simulink model "butterfly_dsp48e_6slice"  (R2012b)
settings: Solver=ode45  StartTime=0.0  StopTime=1999  RelTol=1e-3
libraries: xbsIndex_r4 x255, simulink x8, casper_library_misc x6
(part 1 of 2)
settings Model: Creator=sgowda  LastModifiedBy=sgowda

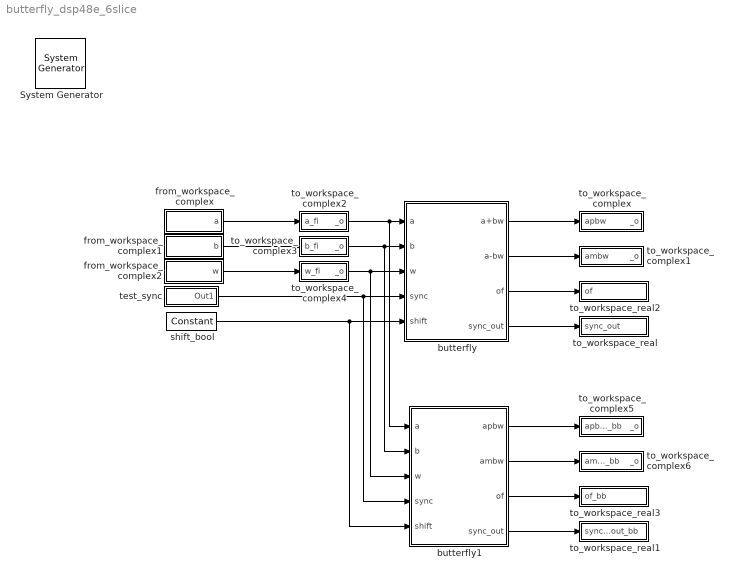
== system butterfly_dsp48e_6slice ==
  " System Generator" : xbsIndex_r4/ System Generator  Tag=genX  xilinxfamily=Kintex7  part=xc7k325t  speed=-3  package=fbg676  synthesis_tool=XST  clock_wrapper=Clock Enables  directory=./netlist  proj_type=Project Navigator  Synth_file=XST Defaults  Impl_file=ISE Defaults  testbench=off  simulink_period=1  sysclk_period=10  dcm_input_clock_period=10  incr_netlist=off  trim_vbits=Everywhere in SubSystem  dbl_ovrd=According to Block Masks  core_generation=According to Block Masks  run_coregen=off  deprecated_control=off  eval_field=0  block_type=sysgen
  butterfly : Subsystem
      settings: AttributesFormatString=|
      | twiddle_general_dsp48e
      | coeffs in slices
      | Bit growth:0
  butterfly1 : Subsystem
  from_workspace_complex : Subsystem  mask{var_name=a, n_bits=18, bin_pt=17, quantization=Truncate, overflow=Wrap, arith_type=Signed  (2's comp)}
      mask prompts: var_name "Workspace variable name"; n_bits "# of bits"; bin_pt "Binary Point"; arith_type "Arithmetic type"
      mask init:
      | config.source = str2func('mat_input_data_cplx_init_xblock');
      | config.toplevel = gcb();
      | xBlock(config, {config.toplevel, 'var_name', var_name, ...
      |     'n_bits', n_bits, 'bin_pt', bin_pt, 'quantization', quantization, ...
      |     'overflow', overflow, 'arith_type', arith_type});
      mask TypeOptions quantization: Truncate | Round  (unbiased: +/- Inf) | Round  (unbiased: Even Values)
      mask TypeOptions overflow: Wrap | Saturate | Flag as error
      mask TypeOptions arith_type: Signed  (2's comp) | Boolean | Unsigned
  from_workspace_complex1 : Subsystem  mask{var_name=b, n_bits=18, bin_pt=17, quantization=Truncate, overflow=Wrap, arith_type=Signed  (2's comp)}
      mask prompts: var_name "Workspace variable name"; n_bits "# of bits"; bin_pt "Binary Point"; arith_type "Arithmetic type"
      mask init: same as butterfly_dsp48e_6slice/from_workspace_complex
      mask TypeOptions quantization: Truncate | Round  (unbiased: +/- Inf) | Round  (unbiased: Even Values)
      mask TypeOptions overflow: Wrap | Saturate | Flag as error
      mask TypeOptions arith_type: Signed  (2's comp) | Boolean | Unsigned
  from_workspace_complex2 : Subsystem  mask{var_name=w, n_bits=18, bin_pt=17, quantization=Truncate, overflow=Wrap, arith_type=Signed  (2's comp)}
      mask prompts: var_name "Workspace variable name"; n_bits "# of bits"; bin_pt "Binary Point"; arith_type "Arithmetic type"
      mask init: same as butterfly_dsp48e_6slice/from_workspace_complex
      mask TypeOptions quantization: Truncate | Round  (unbiased: +/- Inf) | Round  (unbiased: Even Values)
      mask TypeOptions overflow: Wrap | Saturate | Flag as error
      mask TypeOptions arith_type: Signed  (2's comp) | Boolean | Unsigned
  shift_bool : xbsIndex_r4/Constant  const=0  gui_display_data_type=Boolean  arith_type=Boolean  n_bits=32  bin_pt=0  preci_type=Single  exp_width=8  frac_width=24  explicit_period=on  period=1  equ=P=C  opselect=C  inp2=PCIN>>17  opr=+  inp1=P  carry=CIN  dbl_ovrd=off  block_type=constant
  test_sync : Subsystem
  to_workspace_complex : Subsystem  mask{var_name=apbw, n_bits=18, bin_pt=17}
      mask prompts: var_name "Workspace variable name"; n_bits "# of bits"; bin_pt "Binary Point"
      mask init:
      | config.source = str2func('mat_output_data_cplx_init_xblock');
      | config.toplevel = gcb();
      | xBlock(config, {config.toplevel, 'var_name', var_name, ...
      |     'n_bits', n_bits, 'bin_pt', bin_pt})
  to_workspace_complex1 : Subsystem  mask{var_name=ambw, n_bits=18, bin_pt=17}
      mask prompts: var_name "Workspace variable name"; n_bits "# of bits"; bin_pt "Binary Point"
      mask init:
      | config.source = str2func('mat_output_data_cplx_init_xblock');
      | config.toplevel = gcb();
      | xBlock(config, {config.toplevel, 'var_name', var_name, ...
      |     'n_bits', n_bits, 'bin_pt', bin_pt})
  to_workspace_complex2 : Subsystem  mask{var_name=a_fi, n_bits=18, bin_pt=17}
      mask prompts: var_name "Workspace variable name"; n_bits "# of bits"; bin_pt "Binary Point"
      mask init:
      | config.source = str2func('mat_output_data_cplx_init_xblock');
      | config.toplevel = gcb();
      | xBlock(config, {config.toplevel, 'var_name', var_name, ...
      |     'n_bits', n_bits, 'bin_pt', bin_pt});
  to_workspace_complex3 : Subsystem  mask{var_name=b_fi, n_bits=18, bin_pt=17}
      mask prompts: var_name "Workspace variable name"; n_bits "# of bits"; bin_pt "Binary Point"
      mask init:
      | config.source = str2func('mat_output_data_cplx_init_xblock');
      | config.toplevel = gcb();
      | xBlock(config, {config.toplevel, 'var_name', var_name, ...
      |     'n_bits', n_bits, 'bin_pt', bin_pt});
  to_workspace_complex4 : Subsystem  mask{var_name=w_fi, n_bits=18, bin_pt=17}
      mask prompts: var_name "Workspace variable name"; n_bits "# of bits"; bin_pt "Binary Point"
      mask init:
      | config.source = str2func('mat_output_data_cplx_init_xblock');
      | config.toplevel = gcb();
      | xBlock(config, {config.toplevel, 'var_name', var_name, ...
      |     'n_bits', n_bits, 'bin_pt', bin_pt});
  to_workspace_complex5 : Subsystem  mask{var_name=apbw_bb, n_bits=18, bin_pt=17}
      mask prompts: var_name "Workspace variable name"; n_bits "# of bits"; bin_pt "Binary Point"
      mask init:
      | config.source = str2func('mat_output_data_cplx_init_xblock');
      | config.toplevel = gcb();
      | xBlock(config, {config.toplevel, 'var_name', var_name, ...
      |     'n_bits', n_bits, 'bin_pt', bin_pt})
  to_workspace_complex6 : Subsystem  mask{var_name=ambw_bb, n_bits=18, bin_pt=17}
      mask prompts: var_name "Workspace variable name"; n_bits "# of bits"; bin_pt "Binary Point"
      mask init:
      | config.source = str2func('mat_output_data_cplx_init_xblock');
      | config.toplevel = gcb();
      | xBlock(config, {config.toplevel, 'var_name', var_name, ...
      |     'n_bits', n_bits, 'bin_pt', bin_pt})
  to_workspace_real : Subsystem  mask{var_name=sync_out}
      mask prompts: var_name "Workspace variable name"
      mask init:
      | config.source = str2func('mat_output_data_init_xblock');
      | config.toplevel = gcb();
      | xBlock(config, {config.toplevel, 'var_name', var_name});
  to_workspace_real1 : Subsystem  mask{var_name=sync_out_bb}
      mask prompts: var_name "Workspace variable name"
      mask init:
      | config.source = str2func('mat_output_data_init_xblock');
      | config.toplevel = gcb();
      | xBlock(config, {config.toplevel, 'var_name', var_name});
  to_workspace_real2 : Subsystem  mask{var_name=of}
      mask prompts: var_name "Workspace variable name"
      mask init:
      | config.source = str2func('mat_output_data_init_xblock');
      | config.toplevel = gcb();
      | xBlock(config, {config.toplevel, 'var_name', var_name});
  to_workspace_real3 : Subsystem  mask{var_name=of_bb}
      mask prompts: var_name "Workspace variable name"
      mask init:
      | config.source = str2func('mat_output_data_init_xblock');
      | config.toplevel = gcb();
      | xBlock(config, {config.toplevel, 'var_name', var_name});
  wires:
  shift_bool/1 -> butterfly/5(shift), butterfly1/5(shift)
  butterfly/1(a+bw) -> to_workspace_complex/1(apbw)
  butterfly/2(a-bw) -> to_workspace_complex1/1(ambw)
  butterfly/4(sync_out) -> to_workspace_real/1(sync_out)
  butterfly/3(of) -> to_workspace_real2/1(of)
  test_sync/1(Out1) -> butterfly1/4(sync), butterfly/4(sync)
  from_workspace_complex/1(a) -> to_workspace_complex2/1(a_fi)
  from_workspace_complex1/1(b) -> to_workspace_complex3/1(b_fi)
  from_workspace_complex2/1(w) -> to_workspace_complex4/1(w_fi)
  to_workspace_complex2/1(_o) -> butterfly1/1(a), butterfly/1(a)
  to_workspace_complex3/1(_o) -> butterfly1/2(b), butterfly/2(b)
  to_workspace_complex4/1(_o) -> butterfly/3(w), butterfly1/3(w)
  butterfly1/1(apbw) -> to_workspace_complex5/1(apbw_bb)
  butterfly1/2(ambw) -> to_workspace_complex6/1(ambw_bb)
  butterfly1/3(of) -> to_workspace_real3/1(of_bb)
  butterfly1/4(sync_out) -> to_workspace_real1/1(sync_out_bb)

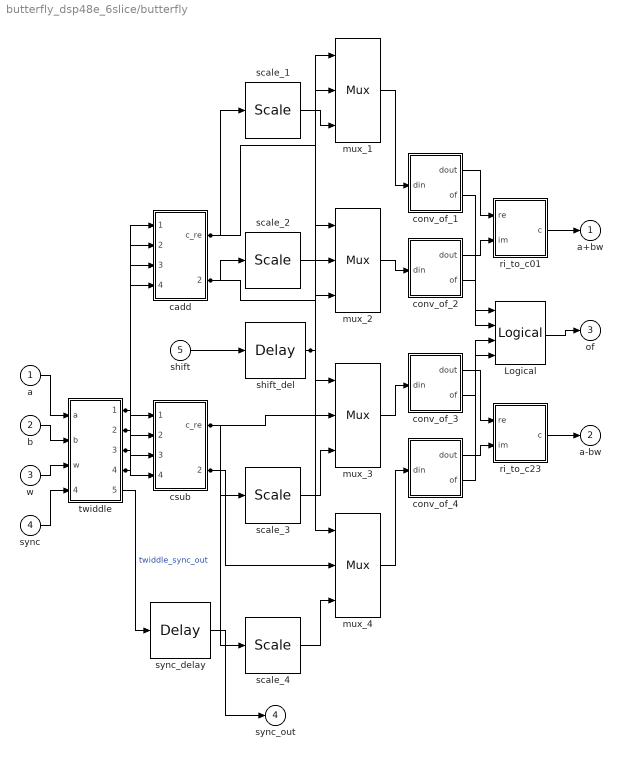
== system butterfly_dsp48e_6slice/butterfly ==
  a : Inport
  b : Inport  Port=2
  w : Inport  Port=3
  sync : Inport  Port=4
  shift : Inport  Port=5
  Logical : xbsIndex_r4/Logical  logical_function=OR  inputs=4  en=off  latency=0  precision=Full  arith_type=Unsigned  n_bits=16  bin_pt=0  align_bp=on  dbl_ovrd=off  block_type=logical
  cadd : Subsystem
  conv_of_1 : Subsystem
      settings: AttributesFormatString=[24,20]->[18,17]
  conv_of_2 : Subsystem
      settings: AttributesFormatString=[24,20]->[18,17]
  conv_of_3 : Subsystem
      settings: AttributesFormatString=[24,20]->[18,17]
  conv_of_4 : Subsystem
      settings: AttributesFormatString=[24,20]->[18,17]
  csub : Subsystem
  mux_{1..4} (4 alike) : xbsIndex_r4/Mux  inputs=2  en=off  latency=1  precision=Full  arith_type=Unsigned  n_bits=16  bin_pt=14  quantization=Truncate  overflow=Wrap  dbl_ovrd=off  block_type=mux
  ri_to_c01 : Subsystem
  ri_to_c23 : Subsystem
  scale_{1..4} (4 alike) : xbsIndex_r4/Scale  scale_factor=-1  dbl_ovrd=off  block_type=scale
  shift_del : xbsIndex_r4/Delay  rst=off  infoeditControl=Selection of Reset will increase slice count due to use of real FFs and instead of SRLs  en=off  latency=2  dbl_ovrd=off  reg_retiming=off  block_type=delay
  sync_delay : xbsIndex_r4/Delay  rst=off  infoeditControl=Selection of Reset will increase slice count due to use of real FFs and instead of SRLs  en=off  latency=4  dbl_ovrd=off  reg_retiming=on  block_type=delay
  twiddle : Subsystem
      settings: AttributesFormatString=|
      | data=(18,17)
      | coeffs=(18,16)
      | Virtex5
      | (Round  (unbiased: +/- Inf),Wrap)
      | twiddle_general_dsp48e
  a+bw : Outport
  a-bw : Outport  Port=2
  of : Outport  Port=3
  sync_out : Outport  Port=4
  wires:
  twiddle/1(a_re) -> csub/1(a_re), cadd/1(a_re)
  twiddle/2(a_im) -> csub/2(a_im), cadd/2(a_im)
  twiddle/3(bw_re) -> csub/3(b_re), cadd/3(b_re)
  twiddle/4(bw_im) -> csub/4(b_im), cadd/4(b_im)
  cadd/1(c_re) -> mux_1/2, scale_1/1
  shift_del/1 -> mux_4/1, mux_3/1, mux_2/1, mux_1/1
  cadd/2(c_im) -> mux_2/2, scale_2/1
  csub/1(c_re) -> mux_3/2, scale_3/1
  csub/2(c_im) -> mux_4/2, scale_4/1
  sync_delay/1 -> sync_out/1
  twiddle/5(sync_out) -> sync_delay/1  "twiddle_sync_out"
  ri_to_c23/1(c) -> a-bw/1
  conv_of_4/1(dout) -> ri_to_c23/2(im)
  conv_of_3/1(dout) -> ri_to_c23/1(re)
  ri_to_c01/1(c) -> a+bw/1
  conv_of_2/1(dout) -> ri_to_c01/2(im)
  conv_of_1/1(dout) -> ri_to_c01/1(re)
  Logical/1 -> of/1
  conv_of_4/2(of) -> Logical/4
  conv_of_3/2(of) -> Logical/3
  conv_of_2/2(of) -> Logical/2
  conv_of_1/2(of) -> Logical/1
  mux_4/1 -> conv_of_4/1(din)
  scale_4/1 -> mux_4/3
  mux_3/1 -> conv_of_3/1(din)
  scale_3/1 -> mux_3/3
  mux_2/1 -> conv_of_2/1(din)
  scale_2/1 -> mux_2/3
  mux_1/1 -> conv_of_1/1(din)
  scale_1/1 -> mux_1/3
  shift/1 -> shift_del/1
  sync/1 -> twiddle/4(sync)
  w/1 -> twiddle/3(w)
  b/1 -> twiddle/2(b)
  a/1 -> twiddle/1(a)

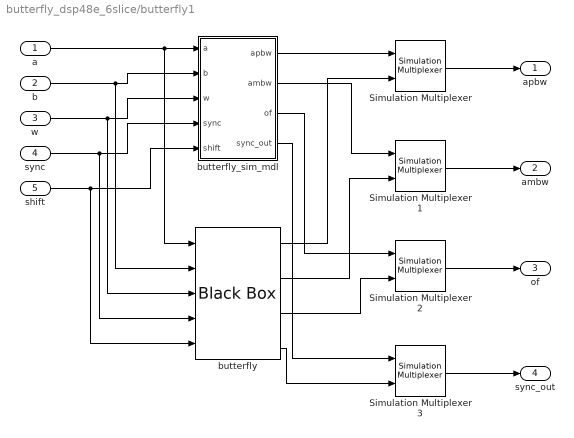
== system butterfly_dsp48e_6slice/butterfly1 ==
  a : Inport
  b : Inport  Port=2
  w : Inport  Port=3
  sync : Inport  Port=4
  shift : Inport  Port=5
  Simulation Multiplexer{,1..3} (4 alike) : xbsIndex_r4/Simulation Multiplexer  sim_sel=1  hw_sel=2  block_type=simmux
      settings: infoedit="Distinguish input subsystems as \"simulation only\" and \"generation only\".  The input specified For Simulation will be used during Simulink simulation.  The input specified For Generation will be used during code generation.  This block will typically be used on the output of a HW Co-Simulation, Black Box, or ModelSim subsystem.<br><br>Hardware Notes: This block costs nothing."
  butterfly : xbsIndex_r4/Black Box  init_code=butterfly_dsp48e_6slice_blackbox_config  sim_method=Inactive  verbose=off  block_type=blackbox2
  butterfly_sim_mdl : Subsystem
  apbw : Outport
  ambw : Outport  Port=2
  of : Outport  Port=3
  sync_out : Outport  Port=4
  wires:
  butterfly/2 -> Simulation Multiplexer1/2
  Simulation Multiplexer1/1 -> ambw/1
  Simulation Multiplexer/1 -> apbw/1
  butterfly_sim_mdl/1(apbw) -> Simulation Multiplexer/1
  butterfly_sim_mdl/3(of) -> Simulation Multiplexer2/1
  butterfly_sim_mdl/2(ambw) -> Simulation Multiplexer1/1
  butterfly/4 -> Simulation Multiplexer3/2
  b/1 -> butterfly/2, butterfly_sim_mdl/2(b)
  a/1 -> butterfly/1, butterfly_sim_mdl/1(a)
  w/1 -> butterfly/3, butterfly_sim_mdl/3(w)
  sync/1 -> butterfly/4, butterfly_sim_mdl/4(sync)
  butterfly/3 -> Simulation Multiplexer2/2
  butterfly_sim_mdl/4(sync_out) -> Simulation Multiplexer3/1
  butterfly/1 -> Simulation Multiplexer/2
  Simulation Multiplexer2/1 -> of/1
  Simulation Multiplexer3/1 -> sync_out/1
  shift/1 -> butterfly/5, butterfly_sim_mdl/5(shift)

== system butterfly_dsp48e_6slice/from_workspace_complex ==
  c_to_ri_simulink : ComplexToRealImag
  gateway_imag : xbsIndex_r4/Gateway In  gui_display_data_type=Fixed-point  arith_type="Signed  (2's comp)"  n_bits=18  bin_pt=17  preci_type=Single  exp_width=8  frac_width=24  quantization=Truncate  overflow=Wrap  period=1  dbl_ovrd=off  timing_constraint=None  locs_specified=off  LOCs={}  UseAsADC=off  ADCChannel='1'  inherit_from_input=off  hdl_port=on  block_type=gatewayin
  gateway_real : xbsIndex_r4/Gateway In  gui_display_data_type=Fixed-point  arith_type="Signed  (2's comp)"  n_bits=18  bin_pt=17  preci_type=Single  exp_width=8  frac_width=24  quantization=Truncate  overflow=Wrap  period=1  dbl_ovrd=off  timing_constraint=None  locs_specified=off  LOCs={}  UseAsADC=off  ADCChannel='1'  inherit_from_input=off  hdl_port=on  block_type=gatewayin
  ri_to_c : Subsystem
  workspace_var : FromWorkspace  VariableName=a  SampleTime=0
  a : Outport
  wires:
  ri_to_c/1(c) -> a/1
  gateway_imag/1 -> ri_to_c/2(im)
  gateway_real/1 -> ri_to_c/1(re)
  c_to_ri_simulink/2 -> gateway_imag/1
  c_to_ri_simulink/1 -> gateway_real/1
  workspace_var/1 -> c_to_ri_simulink/1

== system butterfly_dsp48e_6slice/from_workspace_complex1 ==
  c_to_ri_simulink : ComplexToRealImag
  gateway_imag : xbsIndex_r4/Gateway In  gui_display_data_type=Fixed-point  arith_type="Signed  (2's comp)"  n_bits=18  bin_pt=17  preci_type=Single  exp_width=8  frac_width=24  quantization=Truncate  overflow=Wrap  period=1  dbl_ovrd=off  timing_constraint=None  locs_specified=off  LOCs={}  UseAsADC=off  ADCChannel='1'  inherit_from_input=off  hdl_port=on  block_type=gatewayin
  gateway_real : xbsIndex_r4/Gateway In  gui_display_data_type=Fixed-point  arith_type="Signed  (2's comp)"  n_bits=18  bin_pt=17  preci_type=Single  exp_width=8  frac_width=24  quantization=Truncate  overflow=Wrap  period=1  dbl_ovrd=off  timing_constraint=None  locs_specified=off  LOCs={}  UseAsADC=off  ADCChannel='1'  inherit_from_input=off  hdl_port=on  block_type=gatewayin
  ri_to_c : Subsystem
  workspace_var : FromWorkspace  VariableName=b  SampleTime=0
  b : Outport
  wires:
  ri_to_c/1(c) -> b/1
  gateway_imag/1 -> ri_to_c/2(im)
  gateway_real/1 -> ri_to_c/1(re)
  c_to_ri_simulink/2 -> gateway_imag/1
  c_to_ri_simulink/1 -> gateway_real/1
  workspace_var/1 -> c_to_ri_simulink/1

== system butterfly_dsp48e_6slice/from_workspace_complex2 ==
  c_to_ri_simulink : ComplexToRealImag
  gateway_imag : xbsIndex_r4/Gateway In  gui_display_data_type=Fixed-point  arith_type="Signed  (2's comp)"  n_bits=18  bin_pt=17  preci_type=Single  exp_width=8  frac_width=24  quantization=Truncate  overflow=Wrap  period=1  dbl_ovrd=off  timing_constraint=None  locs_specified=off  LOCs={}  UseAsADC=off  ADCChannel='1'  inherit_from_input=off  hdl_port=on  block_type=gatewayin
  gateway_real : xbsIndex_r4/Gateway In  gui_display_data_type=Fixed-point  arith_type="Signed  (2's comp)"  n_bits=18  bin_pt=17  preci_type=Single  exp_width=8  frac_width=24  quantization=Truncate  overflow=Wrap  period=1  dbl_ovrd=off  timing_constraint=None  locs_specified=off  LOCs={}  UseAsADC=off  ADCChannel='1'  inherit_from_input=off  hdl_port=on  block_type=gatewayin
  ri_to_c : Subsystem
  workspace_var : FromWorkspace  VariableName=w  SampleTime=0
  w : Outport
  wires:
  ri_to_c/1(c) -> w/1
  gateway_imag/1 -> ri_to_c/2(im)
  gateway_real/1 -> ri_to_c/1(re)
  c_to_ri_simulink/2 -> gateway_imag/1
  c_to_ri_simulink/1 -> gateway_real/1
  workspace_var/1 -> c_to_ri_simulink/1

== system butterfly_dsp48e_6slice/test_sync ==
  Constant1 : xbsIndex_r4/Constant  const=1  gui_display_data_type=Boolean  arith_type=Boolean  n_bits=16  bin_pt=14  preci_type=Single  exp_width=8  frac_width=24  explicit_period=on  period=1  equ=P=C  opselect=C  inp2=PCIN>>17  opr=+  inp1=P  carry=CIN  dbl_ovrd=off  block_type=constant
  edge_detect : casper_library_misc/edge_detect  edge=Rising  polarity=Active High  x_in=[0 0.08 0.08 0.16 0.16 0.24 0.24 0.32 0.32 0.4]  y_in="[-1 -1  1  1  1  1  1  1  1  1]"  x_out=[0.6 0.68 0.68 0.76 0.76 0.84 0.84 0.92 0.92 1]  y_out="[-1 -1  1  1 -1 -1 -1 -1 -1 -1]"
  Out1 : Outport
  wires:
  edge_detect/1 -> Out1/1
  Constant1/1 -> edge_detect/1

== system butterfly_dsp48e_6slice/to_workspace_complex ==
  apbw : Inport
  c_to_ri : Subsystem
  imag_gateway : xbsIndex_r4/Gateway Out  inherit_from_input=on  hdl_port=off  timing_constraint=None  locs_specified=off  LOCs={}  UseAsDAC=off  DACChannel='1'  block_type=gatewayout
  real_gateway : xbsIndex_r4/Gateway Out  inherit_from_input=on  hdl_port=off  timing_constraint=None  locs_specified=off  LOCs={}  UseAsDAC=off  DACChannel='1'  block_type=gatewayout
  ri_to_c : RealImagToComplex
  workspace_output : ToWorkspace  VariableName=apbw  SampleTime=-1
  _o : Outport
  wires:
  apbw/1 -> c_to_ri/1(c), _o/1
  ri_to_c/1 -> workspace_output/1  "cplx"
  imag_gateway/1 -> ri_to_c/2
  real_gateway/1 -> ri_to_c/1
  c_to_ri/2(im) -> imag_gateway/1  "c_to_ri_out2"
  c_to_ri/1(re) -> real_gateway/1  "c_to_ri_out1"

== system butterfly_dsp48e_6slice/to_workspace_complex1 ==
  ambw : Inport
  c_to_ri : Subsystem
  imag_gateway : xbsIndex_r4/Gateway Out  inherit_from_input=on  hdl_port=off  timing_constraint=None  locs_specified=off  LOCs={}  UseAsDAC=off  DACChannel='1'  block_type=gatewayout
  real_gateway : xbsIndex_r4/Gateway Out  inherit_from_input=on  hdl_port=off  timing_constraint=None  locs_specified=off  LOCs={}  UseAsDAC=off  DACChannel='1'  block_type=gatewayout
  ri_to_c : RealImagToComplex
  workspace_output : ToWorkspace  VariableName=ambw  SampleTime=-1
  _o : Outport
  wires:
  ambw/1 -> c_to_ri/1(c), _o/1
  ri_to_c/1 -> workspace_output/1  "cplx"
  imag_gateway/1 -> ri_to_c/2
  real_gateway/1 -> ri_to_c/1
  c_to_ri/2(im) -> imag_gateway/1  "c_to_ri_out2"
  c_to_ri/1(re) -> real_gateway/1  "c_to_ri_out1"

== system butterfly_dsp48e_6slice/to_workspace_complex2 ==
  a_fi : Inport
  c_to_ri : Subsystem
  imag_gateway : xbsIndex_r4/Gateway Out  inherit_from_input=on  hdl_port=off  timing_constraint=None  locs_specified=off  LOCs={}  UseAsDAC=off  DACChannel='1'  block_type=gatewayout
  real_gateway : xbsIndex_r4/Gateway Out  inherit_from_input=on  hdl_port=off  timing_constraint=None  locs_specified=off  LOCs={}  UseAsDAC=off  DACChannel='1'  block_type=gatewayout
  ri_to_c : RealImagToComplex
  workspace_output : ToWorkspace  VariableName=a_fi  SampleTime=-1
  _o : Outport
  wires:
  a_fi/1 -> c_to_ri/1(c), _o/1
  ri_to_c/1 -> workspace_output/1  "cplx"
  imag_gateway/1 -> ri_to_c/2
  real_gateway/1 -> ri_to_c/1
  c_to_ri/2(im) -> imag_gateway/1  "c_to_ri_out2"
  c_to_ri/1(re) -> real_gateway/1  "c_to_ri_out1"

== system butterfly_dsp48e_6slice/to_workspace_complex3 ==
  b_fi : Inport
  c_to_ri : Subsystem
  imag_gateway : xbsIndex_r4/Gateway Out  inherit_from_input=on  hdl_port=off  timing_constraint=None  locs_specified=off  LOCs={}  UseAsDAC=off  DACChannel='1'  block_type=gatewayout
  real_gateway : xbsIndex_r4/Gateway Out  inherit_from_input=on  hdl_port=off  timing_constraint=None  locs_specified=off  LOCs={}  UseAsDAC=off  DACChannel='1'  block_type=gatewayout
  ri_to_c : RealImagToComplex
  workspace_output : ToWorkspace  VariableName=b_fi  SampleTime=-1
  _o : Outport
  wires:
  b_fi/1 -> c_to_ri/1(c), _o/1
  ri_to_c/1 -> workspace_output/1  "cplx"
  imag_gateway/1 -> ri_to_c/2
  real_gateway/1 -> ri_to_c/1
  c_to_ri/2(im) -> imag_gateway/1  "c_to_ri_out2"
  c_to_ri/1(re) -> real_gateway/1  "c_to_ri_out1"

== system butterfly_dsp48e_6slice/to_workspace_complex4 ==
  w_fi : Inport
  c_to_ri : Subsystem
  imag_gateway : xbsIndex_r4/Gateway Out  inherit_from_input=on  hdl_port=off  timing_constraint=None  locs_specified=off  LOCs={}  UseAsDAC=off  DACChannel='1'  block_type=gatewayout
  real_gateway : xbsIndex_r4/Gateway Out  inherit_from_input=on  hdl_port=off  timing_constraint=None  locs_specified=off  LOCs={}  UseAsDAC=off  DACChannel='1'  block_type=gatewayout
  ri_to_c : RealImagToComplex
  workspace_output : ToWorkspace  VariableName=w_fi  SampleTime=-1
  _o : Outport
  wires:
  w_fi/1 -> c_to_ri/1(c), _o/1
  ri_to_c/1 -> workspace_output/1  "cplx"
  imag_gateway/1 -> ri_to_c/2
  real_gateway/1 -> ri_to_c/1
  c_to_ri/2(im) -> imag_gateway/1  "c_to_ri_out2"
  c_to_ri/1(re) -> real_gateway/1  "c_to_ri_out1"

== system butterfly_dsp48e_6slice/to_workspace_complex5 ==
  apbw_bb : Inport
  c_to_ri : Subsystem
  imag_gateway : xbsIndex_r4/Gateway Out  inherit_from_input=on  hdl_port=off  timing_constraint=None  locs_specified=off  LOCs={}  UseAsDAC=off  DACChannel='1'  block_type=gatewayout
  real_gateway : xbsIndex_r4/Gateway Out  inherit_from_input=on  hdl_port=off  timing_constraint=None  locs_specified=off  LOCs={}  UseAsDAC=off  DACChannel='1'  block_type=gatewayout
  ri_to_c : RealImagToComplex
  workspace_output : ToWorkspace  VariableName=apbw_bb  SampleTime=-1
  _o : Outport
  wires:
  apbw_bb/1 -> c_to_ri/1(c), _o/1
  ri_to_c/1 -> workspace_output/1  "cplx"
  imag_gateway/1 -> ri_to_c/2
  real_gateway/1 -> ri_to_c/1
  c_to_ri/2(im) -> imag_gateway/1  "c_to_ri_out2"
  c_to_ri/1(re) -> real_gateway/1  "c_to_ri_out1"

== system butterfly_dsp48e_6slice/to_workspace_complex6 ==
  ambw_bb : Inport
  c_to_ri : Subsystem
  imag_gateway : xbsIndex_r4/Gateway Out  inherit_from_input=on  hdl_port=off  timing_constraint=None  locs_specified=off  LOCs={}  UseAsDAC=off  DACChannel='1'  block_type=gatewayout
  real_gateway : xbsIndex_r4/Gateway Out  inherit_from_input=on  hdl_port=off  timing_constraint=None  locs_specified=off  LOCs={}  UseAsDAC=off  DACChannel='1'  block_type=gatewayout
  ri_to_c : RealImagToComplex
  workspace_output : ToWorkspace  VariableName=ambw_bb  SampleTime=-1
  _o : Outport
  wires:
  ambw_bb/1 -> c_to_ri/1(c), _o/1
  ri_to_c/1 -> workspace_output/1  "cplx"
  imag_gateway/1 -> ri_to_c/2
  real_gateway/1 -> ri_to_c/1
  c_to_ri/2(im) -> imag_gateway/1  "c_to_ri_out2"
  c_to_ri/1(re) -> real_gateway/1  "c_to_ri_out1"

== system butterfly_dsp48e_6slice/to_workspace_real ==
  sync_out : Inport
  gateway : xbsIndex_r4/Gateway Out  inherit_from_input=on  hdl_port=off  timing_constraint=None  locs_specified=off  LOCs={}  UseAsDAC=off  DACChannel='1'  block_type=gatewayout
  workspace_input : ToWorkspace  VariableName=sync_out  SampleTime=-1
  wires:
  gateway/1 -> workspace_input/1
  sync_out/1 -> gateway/1

== system butterfly_dsp48e_6slice/to_workspace_real1 ==
  sync_out_bb : Inport
  gateway : xbsIndex_r4/Gateway Out  inherit_from_input=on  hdl_port=off  timing_constraint=None  locs_specified=off  LOCs={}  UseAsDAC=off  DACChannel='1'  block_type=gatewayout
  workspace_input : ToWorkspace  VariableName=sync_out_bb  SampleTime=-1
  wires:
  gateway/1 -> workspace_input/1
  sync_out_bb/1 -> gateway/1

== system butterfly_dsp48e_6slice/to_workspace_real2 ==
  of : Inport
  gateway : xbsIndex_r4/Gateway Out  inherit_from_input=on  hdl_port=off  timing_constraint=None  locs_specified=off  LOCs={}  UseAsDAC=off  DACChannel='1'  block_type=gatewayout
  workspace_input : ToWorkspace  VariableName=of  SampleTime=-1
  wires:
  gateway/1 -> workspace_input/1
  of/1 -> gateway/1

== system butterfly_dsp48e_6slice/to_workspace_real3 ==
  of_bb : Inport
  gateway : xbsIndex_r4/Gateway Out  inherit_from_input=on  hdl_port=off  timing_constraint=None  locs_specified=off  LOCs={}  UseAsDAC=off  DACChannel='1'  block_type=gatewayout
  workspace_input : ToWorkspace  VariableName=of_bb  SampleTime=-1
  wires:
  gateway/1 -> workspace_input/1
  of_bb/1 -> gateway/1

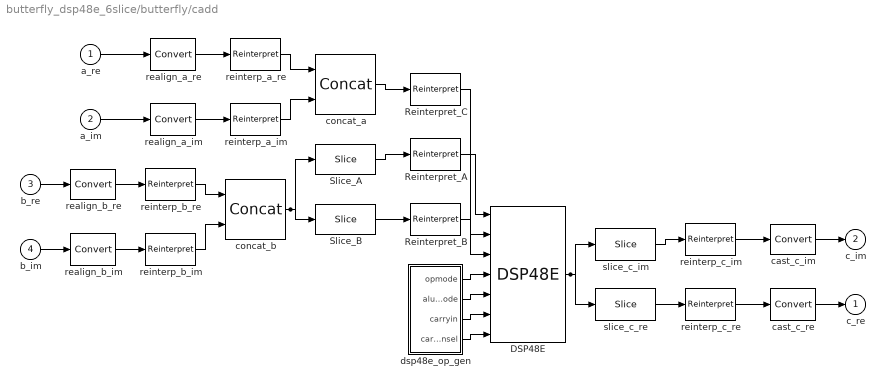
== system butterfly_dsp48e_6slice/butterfly/cadd ==
  a_re : Inport
  a_im : Inport  Port=2
  b_re : Inport  Port=3
  b_im : Inport  Port=4
  DSP48E : xbsIndex_r4/DSP48E  use_a=Direct from A Port  use_b=Direct from B Port  reset_preg=off  pattern_from_creg=on  pattern='000000000000'  mask_from_creg=on  pattern_mask='000000000000'  sel_rounding_mask=Select mask  use_op=off  use_creg=on  rst_all=off  en_all=off  use_pcin=off  use_carrycascin=off  use_multsignin=off  use_carryout=off  use_patterndetect=off  use_patternbdetect=off  use_overflow=off  use_underflow=off  use_acout=off  use_bcout=off  use_pcout=off  use_multsignout=off  use_carrycascout=off  pipeline_a=1  pipeline_b=1  pipeline_acout=1  pipeline_bcout=1  pipeline_c=on  pipeline_p=on  pipeline_mult=on  pipeline_opmode=on  pipeline_alumode=on  pipeline_carryin=on  pipeline_carryinsel=on  rst_a=off  rst_b=off  rst_c=off  rst_mult=off  rst_p=off  rst_carry_in=off  rst_alumode=off  rst_ctrl=off  en_a1=off  en_a2=off  en_b1=off  en_b2=off  en_c=off  en_mult=off  en_p=off  en_carry_in=off  en_alumode=off  en_multcarryin=off  en_ctrl=off  use_synth_model=off  addsub_mode=ONE48  xl_useadderonly=off  block_type=dsp48e
  Reinterpret_A : xbsIndex_r4/Reinterpret  force_arith_type=on  arith_type="Signed  (2's comp)"  force_bin_pt=on  bin_pt=0  block_type=reinterpret
  Reinterpret_B : xbsIndex_r4/Reinterpret  force_arith_type=on  arith_type="Signed  (2's comp)"  force_bin_pt=on  bin_pt=0  block_type=reinterpret
  Reinterpret_C : xbsIndex_r4/Reinterpret  force_arith_type=on  arith_type="Signed  (2's comp)"  force_bin_pt=on  bin_pt=0  block_type=reinterpret
  Slice_A : xbsIndex_r4/Slice  nbits=30  boolean_output=off  mode=Upper Bit Location + Width  bit1=0  base1=MSB of Input  bit0=0  base0=LSB of Input  dbl_ovrd=off  block_type=slice
  Slice_B : xbsIndex_r4/Slice  nbits=18  boolean_output=off  mode=Lower Bit Location + Width  bit1=0  base1=MSB of Input  bit0=0  base0=LSB of Input  dbl_ovrd=off  block_type=slice
  cast_c_im : xbsIndex_r4/Convert  gui_display_data_type=Fixed-point  arith_type="Signed  (2's comp)"  n_bits=23  bin_pt=19  float_type=Single  exp_bits=8  fraction_bits=24  quantization=Truncate  overflow=Wrap  en=off  latency=0  dbl_ovrd=off  pipeline=on  block_type=convert
  cast_c_re : xbsIndex_r4/Convert  gui_display_data_type=Fixed-point  arith_type="Signed  (2's comp)"  n_bits=23  bin_pt=19  float_type=Single  exp_bits=8  fraction_bits=24  quantization=Truncate  overflow=Wrap  en=off  latency=0  dbl_ovrd=off  pipeline=on  block_type=convert
  concat_a : xbsIndex_r4/Concat  num_inputs=2  dbl_ovrd=off  block_type=concat
  concat_b : xbsIndex_r4/Concat  num_inputs=2  dbl_ovrd=off  block_type=concat
  dsp48e_op_gen : Subsystem
  realign_a_im : xbsIndex_r4/Convert  gui_display_data_type=Fixed-point  arith_type="Signed  (2's comp)"  n_bits=24  bin_pt=19  float_type=Single  exp_bits=8  fraction_bits=24  quantization=Truncate  overflow=Wrap  en=off  latency=0  dbl_ovrd=off  pipeline=on  block_type=convert
  realign_a_re : xbsIndex_r4/Convert  gui_display_data_type=Fixed-point  arith_type="Signed  (2's comp)"  n_bits=24  bin_pt=19  float_type=Single  exp_bits=8  fraction_bits=24  quantization=Truncate  overflow=Wrap  en=off  latency=0  dbl_ovrd=off  pipeline=on  block_type=convert
  realign_b_im : xbsIndex_r4/Convert  gui_display_data_type=Fixed-point  arith_type="Signed  (2's comp)"  n_bits=24  bin_pt=19  float_type=Single  exp_bits=8  fraction_bits=24  quantization=Truncate  overflow=Wrap  en=off  latency=0  dbl_ovrd=off  pipeline=on  block_type=convert
  realign_b_re : xbsIndex_r4/Convert  gui_display_data_type=Fixed-point  arith_type="Signed  (2's comp)"  n_bits=24  bin_pt=19  float_type=Single  exp_bits=8  fraction_bits=24  quantization=Truncate  overflow=Wrap  en=off  latency=0  dbl_ovrd=off  pipeline=on  block_type=convert
  reinterp_a_im : xbsIndex_r4/Reinterpret  force_arith_type=on  arith_type=Unsigned  force_bin_pt=on  bin_pt=0  block_type=reinterpret
  reinterp_a_re : xbsIndex_r4/Reinterpret  force_arith_type=on  arith_type=Unsigned  force_bin_pt=on  bin_pt=0  block_type=reinterpret
  reinterp_b_im : xbsIndex_r4/Reinterpret  force_arith_type=on  arith_type=Unsigned  force_bin_pt=on  bin_pt=0  block_type=reinterpret
  reinterp_b_re : xbsIndex_r4/Reinterpret  force_arith_type=on  arith_type=Unsigned  force_bin_pt=on  bin_pt=0  block_type=reinterpret
  reinterp_c_im : xbsIndex_r4/Reinterpret  force_arith_type=on  arith_type="Signed  (2's comp)"  force_bin_pt=on  bin_pt=19  block_type=reinterpret
  reinterp_c_re : xbsIndex_r4/Reinterpret  force_arith_type=on  arith_type="Signed  (2's comp)"  force_bin_pt=on  bin_pt=19  block_type=reinterpret
  slice_c_im : xbsIndex_r4/Slice  nbits=24  boolean_output=off  mode=Lower Bit Location + Width  bit1=0  base1=MSB of Input  bit0=0  base0=LSB of Input  dbl_ovrd=off  block_type=slice
  slice_c_re : xbsIndex_r4/Slice  nbits=24  boolean_output=off  mode=Lower Bit Location + Width  bit1=0  base1=MSB of Input  bit0=24  base0=LSB of Input  dbl_ovrd=off  block_type=slice
  c_re : Outport
  c_im : Outport  Port=2
  wires:
  concat_b/1 -> Slice_B/1, Slice_A/1
  DSP48E/1 -> slice_c_re/1, slice_c_im/1
  slice_c_re/1 -> reinterp_c_re/1
  slice_c_im/1 -> reinterp_c_im/1
  reinterp_c_re/1 -> cast_c_re/1
  reinterp_c_im/1 -> cast_c_im/1
  reinterp_b_re/1 -> concat_b/1
  realign_b_re/1 -> reinterp_b_re/1
  reinterp_b_im/1 -> concat_b/2
  realign_b_im/1 -> reinterp_b_im/1
  reinterp_a_re/1 -> concat_a/1
  realign_a_re/1 -> reinterp_a_re/1
  reinterp_a_im/1 -> concat_a/2
  realign_a_im/1 -> reinterp_a_im/1
  b_re/1 -> realign_b_re/1
  b_im/1 -> realign_b_im/1
  a_re/1 -> realign_a_re/1
  a_im/1 -> realign_a_im/1
  concat_a/1 -> Reinterpret_C/1
  cast_c_re/1 -> c_re/1
  cast_c_im/1 -> c_im/1
  dsp48e_op_gen/4(carryinsel) -> DSP48E/7
  dsp48e_op_gen/3(carryin) -> DSP48E/6
  dsp48e_op_gen/2(alumode) -> DSP48E/5
  dsp48e_op_gen/1(opmode) -> DSP48E/4
  Slice_B/1 -> Reinterpret_B/1
  Slice_A/1 -> Reinterpret_A/1
  Reinterpret_C/1 -> DSP48E/3
  Reinterpret_B/1 -> DSP48E/2
  Reinterpret_A/1 -> DSP48E/1

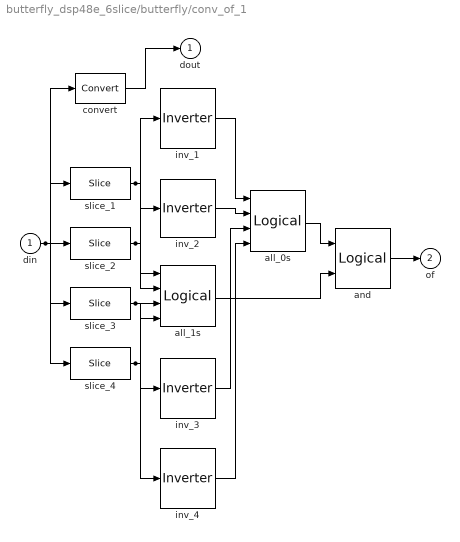
== system butterfly_dsp48e_6slice/butterfly/conv_of_1 ==
  din : Inport
  all_0s : xbsIndex_r4/Logical  logical_function=NAND  inputs=4  en=off  latency=1  precision=Full  arith_type=Unsigned  n_bits=16  bin_pt=0  align_bp=on  dbl_ovrd=off  block_type=logical
  all_1s : xbsIndex_r4/Logical  logical_function=NAND  inputs=4  en=off  latency=1  precision=Full  arith_type=Unsigned  n_bits=16  bin_pt=0  align_bp=on  dbl_ovrd=off  block_type=logical
  and : xbsIndex_r4/Logical  logical_function=AND  inputs=2  en=off  latency=0  precision=Full  arith_type=Unsigned  n_bits=16  bin_pt=0  align_bp=on  dbl_ovrd=off  block_type=logical
  convert : xbsIndex_r4/Convert  gui_display_data_type=Fixed-point  arith_type="Signed  (2's comp)"  n_bits=18  bin_pt=17  float_type=Single  exp_bits=8  fraction_bits=24  quantization="Round  (unbiased: +/- Inf)"  overflow=Saturate  en=off  latency=1  dbl_ovrd=off  pipeline=on  block_type=convert
  inv_{1..4} (4 alike) : xbsIndex_r4/Inverter  en=off  latency=0  dbl_ovrd=off  block_type=inv
  slice_1 : xbsIndex_r4/Slice  nbits=1  boolean_output=on  mode=Upper Bit Location + Width  bit1=0  base1=MSB of Input  bit0=0  base0=LSB of Input  dbl_ovrd=off  block_type=slice
  slice_2 : xbsIndex_r4/Slice  nbits=1  boolean_output=on  mode=Upper Bit Location + Width  bit1=-1  base1=MSB of Input  bit0=0  base0=LSB of Input  dbl_ovrd=off  block_type=slice
  slice_3 : xbsIndex_r4/Slice  nbits=1  boolean_output=on  mode=Upper Bit Location + Width  bit1=-2  base1=MSB of Input  bit0=0  base0=LSB of Input  dbl_ovrd=off  block_type=slice
  slice_4 : xbsIndex_r4/Slice  nbits=1  boolean_output=on  mode=Upper Bit Location + Width  bit1=-3  base1=MSB of Input  bit0=0  base0=LSB of Input  dbl_ovrd=off  block_type=slice
  dout : Outport
  of : Outport  Port=2
  wires:
  din/1 -> slice_4/1, slice_3/1, slice_2/1, slice_1/1, convert/1
  slice_1/1 -> all_1s/1, inv_1/1
  slice_2/1 -> all_1s/2, inv_2/1
  slice_3/1 -> all_1s/3, inv_3/1
  slice_4/1 -> all_1s/4, inv_4/1
  and/1 -> of/1
  all_1s/1 -> and/2
  all_0s/1 -> and/1
  inv_4/1 -> all_0s/4
  inv_3/1 -> all_0s/3
  inv_2/1 -> all_0s/2
  inv_1/1 -> all_0s/1
  convert/1 -> dout/1

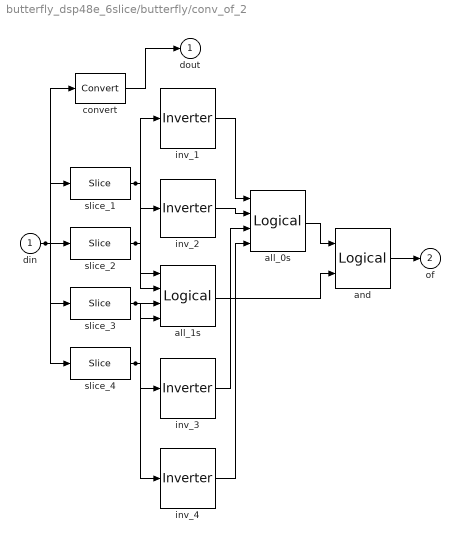
== system butterfly_dsp48e_6slice/butterfly/conv_of_2 ==
  din : Inport
  all_0s : xbsIndex_r4/Logical  logical_function=NAND  inputs=4  en=off  latency=1  precision=Full  arith_type=Unsigned  n_bits=16  bin_pt=0  align_bp=on  dbl_ovrd=off  block_type=logical
  all_1s : xbsIndex_r4/Logical  logical_function=NAND  inputs=4  en=off  latency=1  precision=Full  arith_type=Unsigned  n_bits=16  bin_pt=0  align_bp=on  dbl_ovrd=off  block_type=logical
  and : xbsIndex_r4/Logical  logical_function=AND  inputs=2  en=off  latency=0  precision=Full  arith_type=Unsigned  n_bits=16  bin_pt=0  align_bp=on  dbl_ovrd=off  block_type=logical
  convert : xbsIndex_r4/Convert  gui_display_data_type=Fixed-point  arith_type="Signed  (2's comp)"  n_bits=18  bin_pt=17  float_type=Single  exp_bits=8  fraction_bits=24  quantization="Round  (unbiased: +/- Inf)"  overflow=Saturate  en=off  latency=1  dbl_ovrd=off  pipeline=on  block_type=convert
  inv_{1..4} (4 alike) : xbsIndex_r4/Inverter  en=off  latency=0  dbl_ovrd=off  block_type=inv
  slice_1 : xbsIndex_r4/Slice  nbits=1  boolean_output=on  mode=Upper Bit Location + Width  bit1=0  base1=MSB of Input  bit0=0  base0=LSB of Input  dbl_ovrd=off  block_type=slice
  slice_2 : xbsIndex_r4/Slice  nbits=1  boolean_output=on  mode=Upper Bit Location + Width  bit1=-1  base1=MSB of Input  bit0=0  base0=LSB of Input  dbl_ovrd=off  block_type=slice
  slice_3 : xbsIndex_r4/Slice  nbits=1  boolean_output=on  mode=Upper Bit Location + Width  bit1=-2  base1=MSB of Input  bit0=0  base0=LSB of Input  dbl_ovrd=off  block_type=slice
  slice_4 : xbsIndex_r4/Slice  nbits=1  boolean_output=on  mode=Upper Bit Location + Width  bit1=-3  base1=MSB of Input  bit0=0  base0=LSB of Input  dbl_ovrd=off  block_type=slice
  dout : Outport
  of : Outport  Port=2
  wires:
  din/1 -> slice_4/1, slice_3/1, slice_2/1, slice_1/1, convert/1
  slice_1/1 -> all_1s/1, inv_1/1
  slice_2/1 -> all_1s/2, inv_2/1
  slice_3/1 -> all_1s/3, inv_3/1
  slice_4/1 -> all_1s/4, inv_4/1
  and/1 -> of/1
  all_1s/1 -> and/2
  all_0s/1 -> and/1
  inv_4/1 -> all_0s/4
  inv_3/1 -> all_0s/3
  inv_2/1 -> all_0s/2
  inv_1/1 -> all_0s/1
  convert/1 -> dout/1

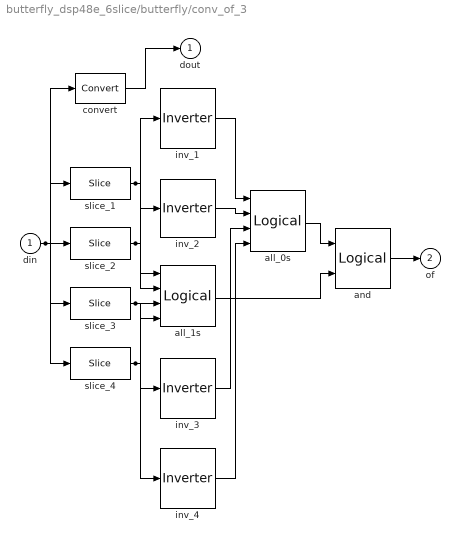
== system butterfly_dsp48e_6slice/butterfly/conv_of_3 ==
  din : Inport
  all_0s : xbsIndex_r4/Logical  logical_function=NAND  inputs=4  en=off  latency=1  precision=Full  arith_type=Unsigned  n_bits=16  bin_pt=0  align_bp=on  dbl_ovrd=off  block_type=logical
  all_1s : xbsIndex_r4/Logical  logical_function=NAND  inputs=4  en=off  latency=1  precision=Full  arith_type=Unsigned  n_bits=16  bin_pt=0  align_bp=on  dbl_ovrd=off  block_type=logical
  and : xbsIndex_r4/Logical  logical_function=AND  inputs=2  en=off  latency=0  precision=Full  arith_type=Unsigned  n_bits=16  bin_pt=0  align_bp=on  dbl_ovrd=off  block_type=logical
  convert : xbsIndex_r4/Convert  gui_display_data_type=Fixed-point  arith_type="Signed  (2's comp)"  n_bits=18  bin_pt=17  float_type=Single  exp_bits=8  fraction_bits=24  quantization="Round  (unbiased: +/- Inf)"  overflow=Saturate  en=off  latency=1  dbl_ovrd=off  pipeline=on  block_type=convert
  inv_{1..4} (4 alike) : xbsIndex_r4/Inverter  en=off  latency=0  dbl_ovrd=off  block_type=inv
  slice_1 : xbsIndex_r4/Slice  nbits=1  boolean_output=on  mode=Upper Bit Location + Width  bit1=0  base1=MSB of Input  bit0=0  base0=LSB of Input  dbl_ovrd=off  block_type=slice
  slice_2 : xbsIndex_r4/Slice  nbits=1  boolean_output=on  mode=Upper Bit Location + Width  bit1=-1  base1=MSB of Input  bit0=0  base0=LSB of Input  dbl_ovrd=off  block_type=slice
  slice_3 : xbsIndex_r4/Slice  nbits=1  boolean_output=on  mode=Upper Bit Location + Width  bit1=-2  base1=MSB of Input  bit0=0  base0=LSB of Input  dbl_ovrd=off  block_type=slice
  slice_4 : xbsIndex_r4/Slice  nbits=1  boolean_output=on  mode=Upper Bit Location + Width  bit1=-3  base1=MSB of Input  bit0=0  base0=LSB of Input  dbl_ovrd=off  block_type=slice
  dout : Outport
  of : Outport  Port=2
  wires:
  din/1 -> slice_4/1, slice_3/1, slice_2/1, slice_1/1, convert/1
  slice_1/1 -> all_1s/1, inv_1/1
  slice_2/1 -> all_1s/2, inv_2/1
  slice_3/1 -> all_1s/3, inv_3/1
  slice_4/1 -> all_1s/4, inv_4/1
  and/1 -> of/1
  all_1s/1 -> and/2
  all_0s/1 -> and/1
  inv_4/1 -> all_0s/4
  inv_3/1 -> all_0s/3
  inv_2/1 -> all_0s/2
  inv_1/1 -> all_0s/1
  convert/1 -> dout/1

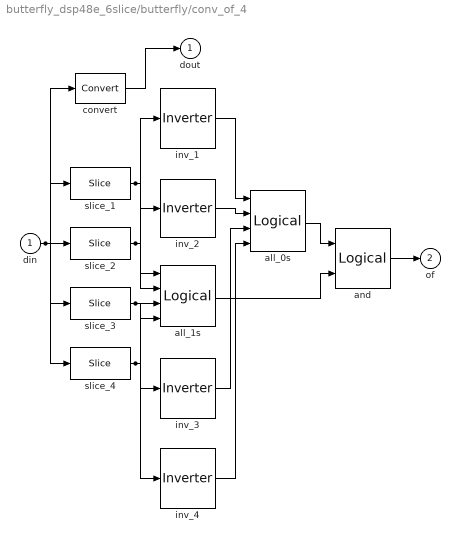
== system butterfly_dsp48e_6slice/butterfly/conv_of_4 ==
  din : Inport
  all_0s : xbsIndex_r4/Logical  logical_function=NAND  inputs=4  en=off  latency=1  precision=Full  arith_type=Unsigned  n_bits=16  bin_pt=0  align_bp=on  dbl_ovrd=off  block_type=logical
  all_1s : xbsIndex_r4/Logical  logical_function=NAND  inputs=4  en=off  latency=1  precision=Full  arith_type=Unsigned  n_bits=16  bin_pt=0  align_bp=on  dbl_ovrd=off  block_type=logical
  and : xbsIndex_r4/Logical  logical_function=AND  inputs=2  en=off  latency=0  precision=Full  arith_type=Unsigned  n_bits=16  bin_pt=0  align_bp=on  dbl_ovrd=off  block_type=logical
  convert : xbsIndex_r4/Convert  gui_display_data_type=Fixed-point  arith_type="Signed  (2's comp)"  n_bits=18  bin_pt=17  float_type=Single  exp_bits=8  fraction_bits=24  quantization="Round  (unbiased: +/- Inf)"  overflow=Saturate  en=off  latency=1  dbl_ovrd=off  pipeline=on  block_type=convert
  inv_{1..4} (4 alike) : xbsIndex_r4/Inverter  en=off  latency=0  dbl_ovrd=off  block_type=inv
  slice_1 : xbsIndex_r4/Slice  nbits=1  boolean_output=on  mode=Upper Bit Location + Width  bit1=0  base1=MSB of Input  bit0=0  base0=LSB of Input  dbl_ovrd=off  block_type=slice
  slice_2 : xbsIndex_r4/Slice  nbits=1  boolean_output=on  mode=Upper Bit Location + Width  bit1=-1  base1=MSB of Input  bit0=0  base0=LSB of Input  dbl_ovrd=off  block_type=slice
  slice_3 : xbsIndex_r4/Slice  nbits=1  boolean_output=on  mode=Upper Bit Location + Width  bit1=-2  base1=MSB of Input  bit0=0  base0=LSB of Input  dbl_ovrd=off  block_type=slice
  slice_4 : xbsIndex_r4/Slice  nbits=1  boolean_output=on  mode=Upper Bit Location + Width  bit1=-3  base1=MSB of Input  bit0=0  base0=LSB of Input  dbl_ovrd=off  block_type=slice
  dout : Outport
  of : Outport  Port=2
  wires:
  din/1 -> slice_4/1, slice_3/1, slice_2/1, slice_1/1, convert/1
  slice_1/1 -> all_1s/1, inv_1/1
  slice_2/1 -> all_1s/2, inv_2/1
  slice_3/1 -> all_1s/3, inv_3/1
  slice_4/1 -> all_1s/4, inv_4/1
  and/1 -> of/1
  all_1s/1 -> and/2
  all_0s/1 -> and/1
  inv_4/1 -> all_0s/4
  inv_3/1 -> all_0s/3
  inv_2/1 -> all_0s/2
  inv_1/1 -> all_0s/1
  convert/1 -> dout/1

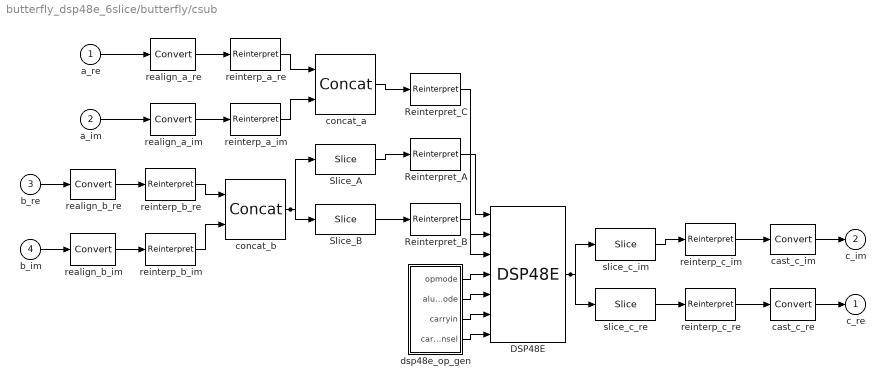
== system butterfly_dsp48e_6slice/butterfly/csub ==
  a_re : Inport
  a_im : Inport  Port=2
  b_re : Inport  Port=3
  b_im : Inport  Port=4
  DSP48E : xbsIndex_r4/DSP48E  use_a=Direct from A Port  use_b=Direct from B Port  reset_preg=off  pattern_from_creg=on  pattern='000000000000'  mask_from_creg=on  pattern_mask='000000000000'  sel_rounding_mask=Select mask  use_op=off  use_creg=on  rst_all=off  en_all=off  use_pcin=off  use_carrycascin=off  use_multsignin=off  use_carryout=off  use_patterndetect=off  use_patternbdetect=off  use_overflow=off  use_underflow=off  use_acout=off  use_bcout=off  use_pcout=off  use_multsignout=off  use_carrycascout=off  pipeline_a=1  pipeline_b=1  pipeline_acout=1  pipeline_bcout=1  pipeline_c=on  pipeline_p=on  pipeline_mult=on  pipeline_opmode=on  pipeline_alumode=on  pipeline_carryin=on  pipeline_carryinsel=on  rst_a=off  rst_b=off  rst_c=off  rst_mult=off  rst_p=off  rst_carry_in=off  rst_alumode=off  rst_ctrl=off  en_a1=off  en_a2=off  en_b1=off  en_b2=off  en_c=off  en_mult=off  en_p=off  en_carry_in=off  en_alumode=off  en_multcarryin=off  en_ctrl=off  use_synth_model=off  addsub_mode=ONE48  xl_useadderonly=off  block_type=dsp48e
  Reinterpret_A : xbsIndex_r4/Reinterpret  force_arith_type=on  arith_type="Signed  (2's comp)"  force_bin_pt=on  bin_pt=0  block_type=reinterpret
  Reinterpret_B : xbsIndex_r4/Reinterpret  force_arith_type=on  arith_type="Signed  (2's comp)"  force_bin_pt=on  bin_pt=0  block_type=reinterpret
  Reinterpret_C : xbsIndex_r4/Reinterpret  force_arith_type=on  arith_type="Signed  (2's comp)"  force_bin_pt=on  bin_pt=0  block_type=reinterpret
  Slice_A : xbsIndex_r4/Slice  nbits=30  boolean_output=off  mode=Upper Bit Location + Width  bit1=0  base1=MSB of Input  bit0=0  base0=LSB of Input  dbl_ovrd=off  block_type=slice
  Slice_B : xbsIndex_r4/Slice  nbits=18  boolean_output=off  mode=Lower Bit Location + Width  bit1=0  base1=MSB of Input  bit0=0  base0=LSB of Input  dbl_ovrd=off  block_type=slice
  cast_c_im : xbsIndex_r4/Convert  gui_display_data_type=Fixed-point  arith_type="Signed  (2's comp)"  n_bits=23  bin_pt=19  float_type=Single  exp_bits=8  fraction_bits=24  quantization=Truncate  overflow=Wrap  en=off  latency=0  dbl_ovrd=off  pipeline=on  block_type=convert
  cast_c_re : xbsIndex_r4/Convert  gui_display_data_type=Fixed-point  arith_type="Signed  (2's comp)"  n_bits=23  bin_pt=19  float_type=Single  exp_bits=8  fraction_bits=24  quantization=Truncate  overflow=Wrap  en=off  latency=0  dbl_ovrd=off  pipeline=on  block_type=convert
  concat_a : xbsIndex_r4/Concat  num_inputs=2  dbl_ovrd=off  block_type=concat
  concat_b : xbsIndex_r4/Concat  num_inputs=2  dbl_ovrd=off  block_type=concat
  dsp48e_op_gen : Subsystem
  realign_a_im : xbsIndex_r4/Convert  gui_display_data_type=Fixed-point  arith_type="Signed  (2's comp)"  n_bits=24  bin_pt=19  float_type=Single  exp_bits=8  fraction_bits=24  quantization=Truncate  overflow=Wrap  en=off  latency=0  dbl_ovrd=off  pipeline=on  block_type=convert
  realign_a_re : xbsIndex_r4/Convert  gui_display_data_type=Fixed-point  arith_type="Signed  (2's comp)"  n_bits=24  bin_pt=19  float_type=Single  exp_bits=8  fraction_bits=24  quantization=Truncate  overflow=Wrap  en=off  latency=0  dbl_ovrd=off  pipeline=on  block_type=convert
  realign_b_im : xbsIndex_r4/Convert  gui_display_data_type=Fixed-point  arith_type="Signed  (2's comp)"  n_bits=24  bin_pt=19  float_type=Single  exp_bits=8  fraction_bits=24  quantization=Truncate  overflow=Wrap  en=off  latency=0  dbl_ovrd=off  pipeline=on  block_type=convert
  realign_b_re : xbsIndex_r4/Convert  gui_display_data_type=Fixed-point  arith_type="Signed  (2's comp)"  n_bits=24  bin_pt=19  float_type=Single  exp_bits=8  fraction_bits=24  quantization=Truncate  overflow=Wrap  en=off  latency=0  dbl_ovrd=off  pipeline=on  block_type=convert
  reinterp_a_im : xbsIndex_r4/Reinterpret  force_arith_type=on  arith_type=Unsigned  force_bin_pt=on  bin_pt=0  block_type=reinterpret
  reinterp_a_re : xbsIndex_r4/Reinterpret  force_arith_type=on  arith_type=Unsigned  force_bin_pt=on  bin_pt=0  block_type=reinterpret
  reinterp_b_im : xbsIndex_r4/Reinterpret  force_arith_type=on  arith_type=Unsigned  force_bin_pt=on  bin_pt=0  block_type=reinterpret
  reinterp_b_re : xbsIndex_r4/Reinterpret  force_arith_type=on  arith_type=Unsigned  force_bin_pt=on  bin_pt=0  block_type=reinterpret
  reinterp_c_im : xbsIndex_r4/Reinterpret  force_arith_type=on  arith_type="Signed  (2's comp)"  force_bin_pt=on  bin_pt=19  block_type=reinterpret
  reinterp_c_re : xbsIndex_r4/Reinterpret  force_arith_type=on  arith_type="Signed  (2's comp)"  force_bin_pt=on  bin_pt=19  block_type=reinterpret
  slice_c_im : xbsIndex_r4/Slice  nbits=24  boolean_output=off  mode=Lower Bit Location + Width  bit1=0  base1=MSB of Input  bit0=0  base0=LSB of Input  dbl_ovrd=off  block_type=slice
  slice_c_re : xbsIndex_r4/Slice  nbits=24  boolean_output=off  mode=Lower Bit Location + Width  bit1=0  base1=MSB of Input  bit0=24  base0=LSB of Input  dbl_ovrd=off  block_type=slice
  c_re : Outport
  c_im : Outport  Port=2
  wires:
  concat_b/1 -> Slice_B/1, Slice_A/1
  DSP48E/1 -> slice_c_re/1, slice_c_im/1
  slice_c_re/1 -> reinterp_c_re/1
  slice_c_im/1 -> reinterp_c_im/1
  reinterp_c_re/1 -> cast_c_re/1
  reinterp_c_im/1 -> cast_c_im/1
  reinterp_b_re/1 -> concat_b/1
  realign_b_re/1 -> reinterp_b_re/1
  reinterp_b_im/1 -> concat_b/2
  realign_b_im/1 -> reinterp_b_im/1
  reinterp_a_re/1 -> concat_a/1
  realign_a_re/1 -> reinterp_a_re/1
  reinterp_a_im/1 -> concat_a/2
  realign_a_im/1 -> reinterp_a_im/1
  b_re/1 -> realign_b_re/1
  b_im/1 -> realign_b_im/1
  a_re/1 -> realign_a_re/1
  a_im/1 -> realign_a_im/1
  concat_a/1 -> Reinterpret_C/1
  cast_c_re/1 -> c_re/1
  cast_c_im/1 -> c_im/1
  dsp48e_op_gen/4(carryinsel) -> DSP48E/7
  dsp48e_op_gen/3(carryin) -> DSP48E/6
  dsp48e_op_gen/2(alumode) -> DSP48E/5
  dsp48e_op_gen/1(opmode) -> DSP48E/4
  Slice_B/1 -> Reinterpret_B/1
  Slice_A/1 -> Reinterpret_A/1
  Reinterpret_C/1 -> DSP48E/3
  Reinterpret_B/1 -> DSP48E/2
  Reinterpret_A/1 -> DSP48E/1

== system butterfly_dsp48e_6slice/butterfly/ri_to_c01 ==
  re : Inport
  im : Inport  Port=2
  concat : xbsIndex_r4/Concat  num_inputs=2  dbl_ovrd=off  block_type=concat
  force_im : xbsIndex_r4/Reinterpret  force_arith_type=on  arith_type=Unsigned  force_bin_pt=on  bin_pt=0  block_type=reinterpret
  force_re : xbsIndex_r4/Reinterpret  force_arith_type=on  arith_type=Unsigned  force_bin_pt=on  bin_pt=0  block_type=reinterpret
  c : Outport
  wires:
  force_re/1 -> concat/1
  re/1 -> force_re/1
  force_im/1 -> concat/2
  im/1 -> force_im/1
  concat/1 -> c/1

== system butterfly_dsp48e_6slice/butterfly/ri_to_c23 ==
  re : Inport
  im : Inport  Port=2
  concat : xbsIndex_r4/Concat  num_inputs=2  dbl_ovrd=off  block_type=concat
  force_im : xbsIndex_r4/Reinterpret  force_arith_type=on  arith_type=Unsigned  force_bin_pt=on  bin_pt=0  block_type=reinterpret
  force_re : xbsIndex_r4/Reinterpret  force_arith_type=on  arith_type=Unsigned  force_bin_pt=on  bin_pt=0  block_type=reinterpret
  c : Outport
  wires:
  force_re/1 -> concat/1
  re/1 -> force_re/1
  force_im/1 -> concat/2
  im/1 -> force_im/1
  concat/1 -> c/1

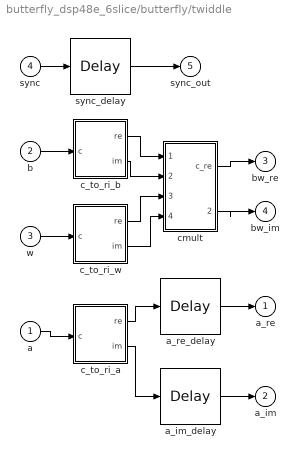
== system butterfly_dsp48e_6slice/butterfly/twiddle ==
  a : Inport
  b : Inport  Port=2
  w : Inport  Port=3
  sync : Inport  Port=4
  a_im_delay : xbsIndex_r4/Delay  rst=off  infoeditControl=Selection of Reset will increase slice count due to use of real FFs and instead of SRLs  en=off  latency=5  dbl_ovrd=off  reg_retiming=on  block_type=delay
  a_re_delay : xbsIndex_r4/Delay  rst=off  infoeditControl=Selection of Reset will increase slice count due to use of real FFs and instead of SRLs  en=off  latency=5  dbl_ovrd=off  reg_retiming=on  block_type=delay
  c_to_ri_a : Subsystem
  c_to_ri_b : Subsystem
  c_to_ri_w : Subsystem
  cmult : Subsystem
  sync_delay : xbsIndex_r4/Delay  rst=off  infoeditControl=Selection of Reset will increase slice count due to use of real FFs and instead of SRLs  en=off  latency=5  dbl_ovrd=off  reg_retiming=off  block_type=delay
  a_re : Outport
  a_im : Outport  Port=2
  bw_re : Outport  Port=3
  bw_im : Outport  Port=4
  sync_out : Outport  Port=5
  wires:
  cmult/2(c_im) -> bw_im/1
  cmult/1(c_re) -> bw_re/1
  c_to_ri_w/2(im) -> cmult/4(b_im)
  c_to_ri_w/1(re) -> cmult/3(b_re)
  c_to_ri_b/2(im) -> cmult/2(a_im)
  c_to_ri_b/1(re) -> cmult/1(a_re)
  a_im_delay/1 -> a_im/1
  c_to_ri_a/2(im) -> a_im_delay/1
  a_re_delay/1 -> a_re/1
  c_to_ri_a/1(re) -> a_re_delay/1
  sync_delay/1 -> sync_out/1
  sync/1 -> sync_delay/1
  w/1 -> c_to_ri_w/1(c)
  b/1 -> c_to_ri_b/1(c)
  a/1 -> c_to_ri_a/1(c)
